simulink library "fam_force_allocation_module_lib"  (R2016b)
settings: Solver=ode45  StartTime=0.0  StopTime=10.0  RelTol=1e-3  EnableMultiTasking=on
values from neighbouring files (symbols this model uses):
  fam_nozzle_orientations = [abp_PM1_nozzle_orientations; abp_PM2_nozzle_orientations]    [fam_force_allocation_module_prep.m]
  fam_P_nozzle_B_B = [abp_PM1_P_nozzle_B_B; abp_PM2_P_nozzle_B_B]    [fam_force_allocation_module_prep.m]
undefined symbols (not defined in the file or in its folder): fam_lookup_thrust_in
libraries: simulink x8, fam_force_allocation_module_lib x2
settings Model: Creator=jfusco1  LastModifiedBy=jfusco1
settings DataIOCC: LimitDataPoints=on  SaveFormat=Array
settings OptimizationCC: LifeSpan=inf
settings DebuggingCC: SolverPrmCheckMsg=warning  AllowSymbolicDim=off  SFUnexpectedBacktrackingDiag=warning  SFNoUnconditionalDefaultTransitionDiag=warning  SFExecutionAtInitializationDiag=none
settings HardwareCC: ProdBitPerPointer=32  ProdBitPerSizeT=32  ProdBitPerPtrDiffT=32  ProdLargestAtomicFloat=None  ProdIntDivRoundTo=Undefined  ProdEndianess=Unspecified  ProdWordSize=32  ProdHWDeviceType=32-bit Generic
settings ModelReferenceCC: PropagateSignalLabelsOutOfModel=off
settings GRTTargetCC: TargetLangStandard=C89/C90 (ANSI)  GeneratePreprocessorConditionals=Disable all
settings ConfigComp: CovMetricSettings=dw  CovHtmlReporting=on  CovSaveCumulativeToWorkspaceVar=on  CovSaveSingleToWorkspaceVar=on  CovExternalEMLEnable=off  CovSFcnEnable=off

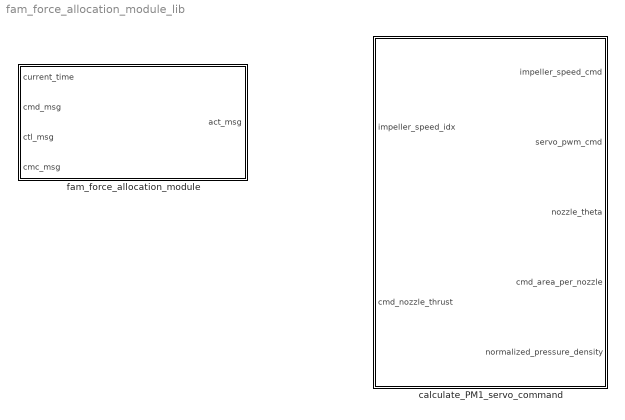
== system fam_force_allocation_module_lib ==
  calculate_PM1_servo_command : Subsystem  mask{impeller_speed_cnt=0, impeller_speeds=0, impeller_speed2pwm=0, impeller_diameter=0, lookup_Cdp=0, lookup_thrust=0, nozzle_widths=0, nozzle_flap_cnt=0, nozzle_flap_length=0, nozzle_in_height=0, nozzle_discharge_coeff=0, nozzle_min_angle=0, nozzle_max_angle=0, nozzle_angle2pwm=0, servo_min_pwm=0, air_density=0}
      mask prompts: impeller_speed_cnt "Number of Speeds"; impeller_speeds "Speeds vs idx"; impeller_speed2pwm "Speed2PWM conversion"; impeller_diameter "Diameter"; lookup_Cdp "Cdp Data"; lookup_thrust "Thrust Breakpoints"; nozzle_widths "Widths"; nozzle_flap_cnt "Flap Count"; nozzle_flap_length "Flap Length"; nozzle_in_height "Intake Height"; nozzle_discharge_coeff "Discharge Coefficients"; nozzle_min_angle "Min Open Angle"; nozzle_max_angle "Max Open Angle"; nozzle_angle2pwm "Angle2PWM conversion"; servo_min_pwm "Minimum PWM"; air_density "Air Density"
      mask DialogControl DescTextVar Prompt: Converts nozzle thrust commands into servo commands
  fam_force_allocation_module : Subsystem

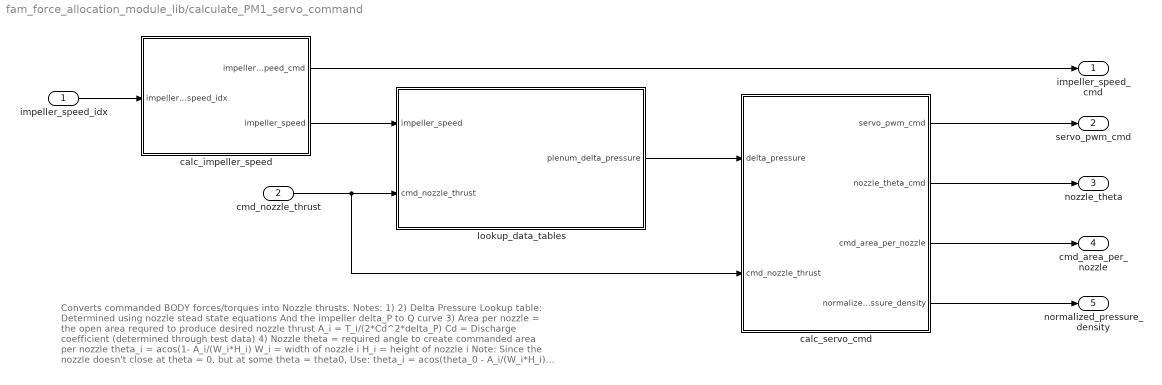
== system fam_force_allocation_module_lib/calculate_PM1_servo_command ==
  note: Converts commanded BODY forces/torques into Nozzle thrusts.
      |
      | Notes:
      | 1)
      | 2) Delta Pressure Lookup table:
      | Determined using nozzle stead state equations
      | And the impeller delta_P to Q curve
      | 3) Area per nozzle = the open area requred to produce desired nozzle thrust
      | A_i = T_i/(2*Cd^2*delta_P)
      | Cd = Discharge coefficient (determined through test data)
      | 4) Nozzle theta = required angle to create commanded area per nozzle
      | theta_i = acos(1- A_i/(W_i*H_i)
      | W_i = width of nozzle i
      | H_i = height of nozzle i
      | Note: Since the nozzle doesn't close at theta = 0, but at some theta = theta0,
      | Use: theta_i = acos(theta_0 - A_i/(W_i*H_i)
      | 5) servo_thetas = commanded theta to each servo
      | theta_si = theta_ni*R
      | R= gear ratio
      | theta_ni = commanded nozzle theta of nozzle 'i'
  impeller_speed_idx : Inport
  cmd_nozzle_thrust : Inport  Port=2
  calc_impeller_speed : Subsystem
  calc_servo_cmd : Subsystem
  lookup_data_tables : Subsystem
  impeller_speed_cmd : Outport
  servo_pwm_cmd : Outport  Port=2
  nozzle_theta : Outport  Port=3
  cmd_area_per_nozzle : Outport  Port=4
  normalized_pressure_density : Outport  Port=5
  wires:
  calc_servo_cmd/4(normalized_pressure_density) -> normalized_pressure_density/1
  calc_servo_cmd/3(cmd_area_per_nozzle) -> cmd_area_per_nozzle/1
  calc_servo_cmd/2(nozzle_theta_cmd) -> nozzle_theta/1
  calc_servo_cmd/1(servo_pwm_cmd) -> servo_pwm_cmd/1
  cmd_nozzle_thrust/1 -> lookup_data_tables/2(cmd_nozzle_thrust), calc_servo_cmd/2(cmd_nozzle_thrust)
  lookup_data_tables/1(plenum_delta_pressure) -> calc_servo_cmd/1(delta_pressure)
  impeller_speed_idx/1 -> calc_impeller_speed/1(impeller_speed_idx)
  calc_impeller_speed/2(impeller_speed) -> lookup_data_tables/1(impeller_speed)
  calc_impeller_speed/1(impeller_speed_cmd) -> impeller_speed_cmd/1

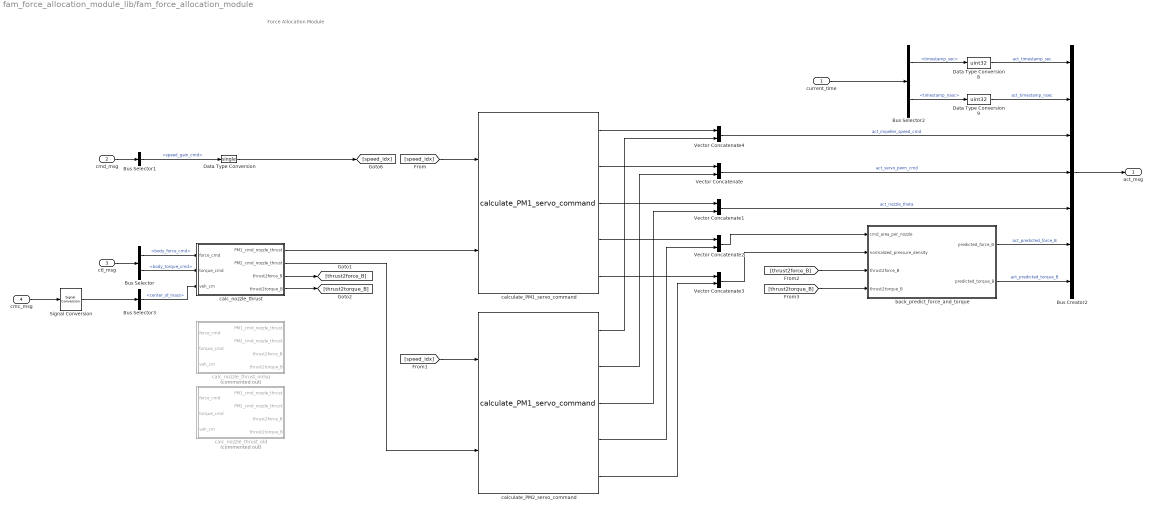
== system fam_force_allocation_module_lib/fam_force_allocation_module ==
  note: Force Allocation Module
  current_time : Inport
  cmd_msg : Inport  Port=2
  ctl_msg : Inport  Port=3
  cmc_msg : Inport  Port=4  OutDataTypeStr=Bus: cmc_msg
  Bus Creator2 : BusCreator  Inputs=7  OutDataTypeStr=Bus: act_msg  NonVirtualBus=on
      settings: InheritFromInputs=off
  Bus Selector : BusSelector  OutputSignals=body_force_cmd,body_torque_cmd
  Bus Selector1 : BusSelector  OutputSignals=speed_gain_cmd
  Bus Selector2 : BusSelector  OutputSignals=timestamp_sec,timestamp_nsec
  Bus Selector3 : BusSelector  OutputSignals=center_of_mass
  Data Type Conversion : DataTypeConversion  OutDataTypeStr=single
  Data Type Conversion8 : DataTypeConversion  OutDataTypeStr=uint32
  Data Type Conversion9 : DataTypeConversion  OutDataTypeStr=uint32
  Signal Conversion : SignalConversion  OverrideOpt=on
  Vector Concatenate{,1..4} (5 alike) : Concatenate
  back_predict_force_and_torque : Subsystem
  calc_nozzle_thrust : Subsystem
  calc_nozzle_thrust_nnlsq : Subsystem  Commented=on
  calc_nozzle_thrust_old : Subsystem  Commented=on
  calculate_PM1_servo_command : fam_force_allocation_module_lib/calculate_PM1_servo_command  impeller_speed_cnt=fam_impeller_speeds_cnt  impeller_speeds=fam_impeller_speeds  impeller_speed2pwm=abp_impeller_speed2pwm  impeller_diameter=abp_impeller_diameter  lookup_Cdp=fam_PM1_lookup_Cdp_data  lookup_thrust=fam_PM1_lookup_thrust_breakpoints  nozzle_widths=abp_PM1_nozzle_widths  nozzle_flap_cnt=abp_nozzle_flap_count  nozzle_flap_length=abp_nozzle_flap_length  nozzle_in_height=abp_nozzle_intake_height  nozzle_discharge_coeff=abp_PM1_discharge_coeff  nozzle_min_angle=abp_nozzle_min_open_angle  nozzle_max_angle=abp_nozzle_max_open_angle  nozzle_angle2pwm=fam_nozzle_angle2pwm  servo_min_pwm=abp_servo_min_PWM  air_density=const_air_density
  calculate_PM2_servo_command : fam_force_allocation_module_lib/calculate_PM1_servo_command  impeller_speed_cnt=fam_impeller_speeds_cnt  impeller_speeds=fam_impeller_speeds  impeller_speed2pwm=abp_impeller_speed2pwm  impeller_diameter=abp_impeller_diameter  lookup_Cdp=fam_PM2_lookup_Cdp_data  lookup_thrust=fam_PM2_lookup_thrust_breakpoints  nozzle_widths=abp_PM2_nozzle_widths  nozzle_flap_cnt=abp_nozzle_flap_count  nozzle_flap_length=abp_nozzle_flap_length  nozzle_in_height=abp_nozzle_intake_height  nozzle_discharge_coeff=abp_PM2_discharge_coeff  nozzle_min_angle=abp_nozzle_min_open_angle  nozzle_max_angle=abp_nozzle_max_open_angle  nozzle_angle2pwm=fam_nozzle_angle2pwm  servo_min_pwm=abp_servo_min_PWM  air_density=const_air_density
  act_msg : Outport
  wires:
  [thrust2torque_B] -> back_predict_force_and_torque/4(thrust2torque_B)
  [thrust2force_B] -> back_predict_force_and_torque/3(thrust2force_B)
  calc_nozzle_thrust/4(thrust2torque_B) -> [thrust2torque_B]
  calc_nozzle_thrust/3(thrust2force_B) -> [thrust2force_B]
  back_predict_force_and_torque/2(predicted_torque_B) -> Bus Creator2/7  "act_predicted_torque_B"
  back_predict_force_and_torque/1(predicted_force_B) -> Bus Creator2/6  "act_predicted_force_B"
  calc_nozzle_thrust/2(PM2_cmd_nozzle_thrust) -> calculate_PM2_servo_command/2
  calc_nozzle_thrust/1(PM1_cmd_nozzle_thrust) -> calculate_PM1_servo_command/2
  [speed_idx] -> calculate_PM2_servo_command/1
  [speed_idx] -> calculate_PM1_servo_command/1
  calculate_PM2_servo_command/5 -> Vector Concatenate3/2
  calculate_PM2_servo_command/4 -> Vector Concatenate2/2
  calculate_PM2_servo_command/3 -> Vector Concatenate1/2
  calculate_PM2_servo_command/2 -> Vector Concatenate/2
  calculate_PM2_servo_command/1 -> Vector Concatenate4/2
  calculate_PM1_servo_command/5 -> Vector Concatenate3/1
  calculate_PM1_servo_command/4 -> Vector Concatenate2/1
  calculate_PM1_servo_command/3 -> Vector Concatenate1/1
  calculate_PM1_servo_command/2 -> Vector Concatenate/1
  calculate_PM1_servo_command/1 -> Vector Concatenate4/1
  Vector Concatenate3/1 -> back_predict_force_and_torque/2(normalized_pressure_density)
  Vector Concatenate2/1 -> back_predict_force_and_torque/1(cmd_area_per_nozzle)
  Vector Concatenate1/1 -> Bus Creator2/5  "act_nozzle_theta"
  Vector Concatenate/1 -> Bus Creator2/4  "act_servo_pwm_cmd"
  Data Type Conversion/1 -> [speed_idx]
  Vector Concatenate4/1 -> Bus Creator2/3  "act_impeller_speed_cmd"
  Data Type Conversion8/1 -> Bus Creator2/1  "act_timestamp_sec"
  Data Type Conversion9/1 -> Bus Creator2/2  "act_timestamp_nsec"
  Bus Selector2/1 -> Data Type Conversion8/1  "<timestamp_sec>"
  Bus Selector2/2 -> Data Type Conversion9/1  "<timestamp_nsec>"
  Bus Creator2/1 -> act_msg/1
  current_time/1 -> Bus Selector2/1
  Bus Selector/2 -> calc_nozzle_thrust/2(torque_cmd)  "<body_torque_cmd>"
  Bus Selector/1 -> calc_nozzle_thrust/1(force_cmd)  "<body_force_cmd>"
  ctl_msg/1 -> Bus Selector/1
  cmd_msg/1 -> Bus Selector1/1
  Bus Selector1/1 -> Data Type Conversion/1  "<speed_gain_cmd>"
  Signal Conversion/1 -> Bus Selector3/1
  Bus Selector3/1 -> calc_nozzle_thrust/3(veh_cm)  "<center_of_mass>"
  cmc_msg/1 -> Signal Conversion/1

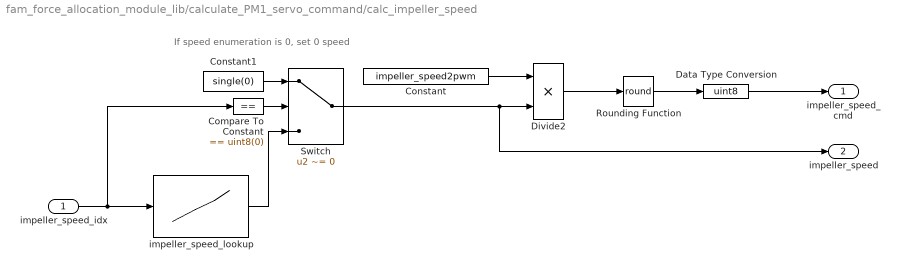
== system fam_force_allocation_module_lib/calculate_PM1_servo_command/calc_impeller_speed ==
  note: If speed enumeration is 0, set 0 speed
  impeller_speed_idx : Inport
  Compare To Constant : simulink/Logic and Bit Operations/Compare To Constant  relop===  const=uint8(0)  OutDataTypeStr=boolean
  Constant : Constant  Value=impeller_speed2pwm
  Constant1 : Constant  Value=single(0)
  Data Type Conversion : DataTypeConversion  OutDataTypeStr=uint8
  Divide2 : Product  Inputs=**
  Rounding Function : Rounding  Operator=round
  Switch : Switch  Criteria=u2 ~= 0
  impeller_speed_lookup : Lookup_n-D  NumberOfTableDimensions=1  BreakpointsForDimension1=[1:impeller_speed_cnt]  BreakpointsForDimension2=fam_lookup_thrust_in  BeginIndexSearchUsingPreviousIndexResult=on  Table=impeller_speeds  InterpMethod=Nearest  ExtrapMethod=Clip  InternalRulePriority=Speed  RndMeth=Simplest  InputSameDT=on
      settings: AttributesFormatString=|
      | Data Table: %<Table>
      | #dim: %<NumberOfTableDimensions>
      | BP1: %<BreakpointsForDimension1>
  impeller_speed_cmd : Outport
  impeller_speed : Outport  Port=2
  wires:
  Data Type Conversion/1 -> impeller_speed_cmd/1
  Rounding Function/1 -> Data Type Conversion/1
  Divide2/1 -> Rounding Function/1
  Constant/1 -> Divide2/1
  impeller_speed_idx/1 -> impeller_speed_lookup/1, Compare To Constant/1
  Switch/1 -> impeller_speed/1, Divide2/2
  Compare To Constant/1 -> Switch/2
  Constant1/1 -> Switch/1
  impeller_speed_lookup/1 -> Switch/3

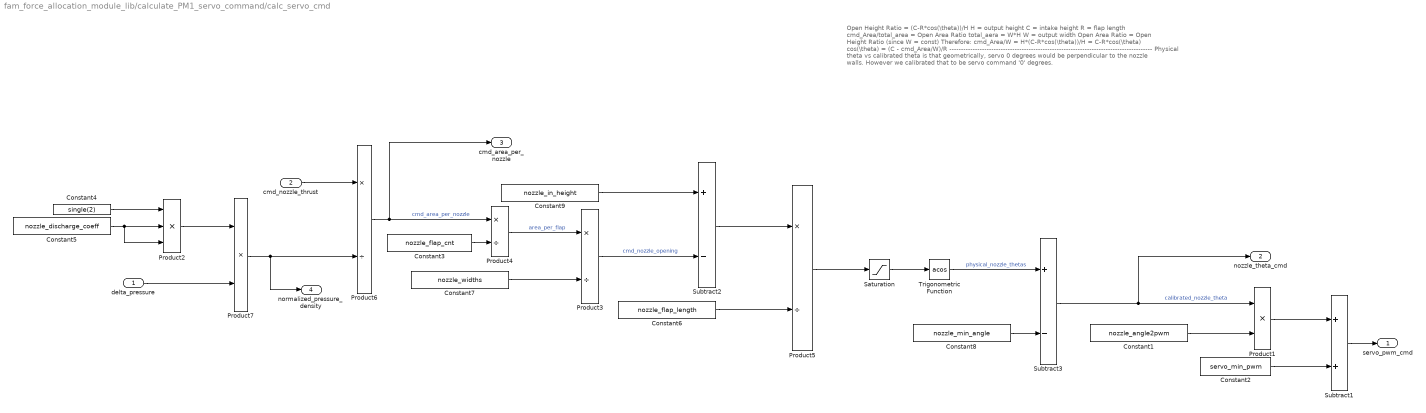
== system fam_force_allocation_module_lib/calculate_PM1_servo_command/calc_servo_cmd ==
  note: Open Height Ratio = (C-R*cos(\theta))/H
      | 	H = output height
      | 	C = intake height
      | 	R = flap length
      |
      | cmd_Area/total_area = Open Area Ratio
      | 	total_aera = W*H
      | 	W = output width
      |
      | Open Area Ratio = Open Height Ratio (since W = const)
      |
      | Therefore:
      | cmd_Area/W = H*(C-R*cos(\theta))/H = C-R*cos(\theta)
      | cos(\theta) = (C - cmd_Area/W)/R
      |
      | ---------------------------------------------------------------------------------------
      |
      | Physical theta vs calibrated theta is that geometrically, servo 0 degrees would be perpendicular to the nozzle walls.
      | 	However we calibrated that to be servo command '0' degrees.
  delta_pressure : Inport
  cmd_nozzle_thrust : Inport  Port=2
  Constant1 : Constant  Value=nozzle_angle2pwm
  Constant2 : Constant  Value=servo_min_pwm
  Constant3 : Constant  Value=nozzle_flap_cnt
  Constant4 : Constant  Value=single(2)
  Constant5 : Constant  Value=nozzle_discharge_coeff
  Constant6 : Constant  Value=nozzle_flap_length
  Constant7 : Constant  Value=nozzle_widths
  Constant8 : Constant  Value=nozzle_min_angle
  Constant9 : Constant  Value=nozzle_in_height
  Product1 : Product  Inputs=**
  Product2 : Product  Inputs=***
  Product{3..6} (4 alike) : Product  Inputs=*/
  Product7 : Product  Inputs=**
  Saturation : Saturate  UpperLimit=cos(nozzle_min_angle)  LowerLimit=cos(nozzle_max_angle)
      settings: AttributesFormatString=|
      | Max: %<UpperLimit>
      | Min: %<LowerLimit>
  Subtract1 : Sum
  Subtract2 : Sum  Inputs=+-
  Subtract3 : Sum  Inputs=+-
  Trigonometric Function : Trigonometry  Operator=acos
  servo_pwm_cmd : Outport
  nozzle_theta_cmd : Outport  Port=2
  cmd_area_per_nozzle : Outport  Port=3
  normalized_pressure_density : Outport  Port=4
  wires:
  Saturation/1 -> Trigonometric Function/1
  Product5/1 -> Saturation/1
  Product6/1 -> cmd_area_per_nozzle/1, Product4/1  "cmd_area_per_nozzle"
  Constant4/1 -> Product2/1
  Product1/1 -> Subtract1/1
  Subtract1/1 -> servo_pwm_cmd/1
  Constant1/1 -> Product1/2
  Constant2/1 -> Subtract1/2
  Constant5/1 -> Product2/3, Product2/2
  delta_pressure/1 -> Product7/2
  Product2/1 -> Product7/1
  Constant7/1 -> Product3/2
  Product3/1 -> Subtract2/2  "cmd_nozzle_opening"
  Constant9/1 -> Subtract2/1
  Constant6/1 -> Product5/2
  Subtract2/1 -> Product5/1
  Constant3/1 -> Product4/2
  Product4/1 -> Product3/1  "area_per_flap"
  Product7/1 -> Product6/2, normalized_pressure_density/1
  cmd_nozzle_thrust/1 -> Product6/1
  Trigonometric Function/1 -> Subtract3/1  "physical_nozzle_thetas"
  Subtract3/1 -> Product1/1, nozzle_theta_cmd/1  "calibrated_nozzle_theta"
  Constant8/1 -> Subtract3/2

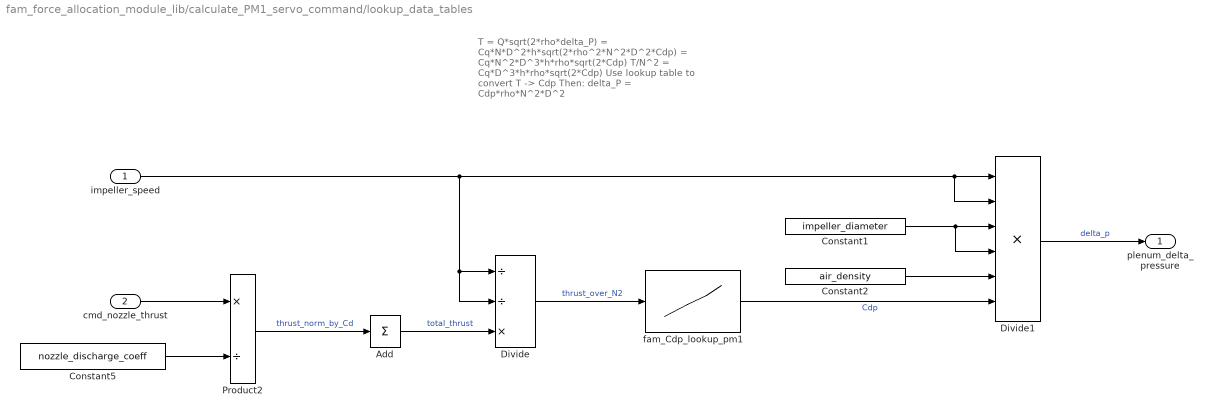
== system fam_force_allocation_module_lib/calculate_PM1_servo_command/lookup_data_tables ==
  note: T = Q*sqrt(2*rho*delta_P)
      | 	= Cq*N*D^2*h*sqrt(2*rho^2*N^2*D^2*Cdp)
      | 	= Cq*N^2*D^3*h*rho*sqrt(2*Cdp)
      | T/N^2 = Cq*D^3*h*rho*sqrt(2*Cdp)
      |
      | Use lookup table to convert T -> Cdp
      | Then: delta_P = Cdp*rho*N^2*D^2
  impeller_speed : Inport
  cmd_nozzle_thrust : Inport  Port=2
  Add : Sum  Inputs=+
  Constant1 : Constant  Value=impeller_diameter
  Constant2 : Constant  Value=air_density
  Constant5 : Constant  Value=nozzle_discharge_coeff
  Divide : Product  Inputs=//*
  Divide1 : Product  Inputs=******
  Product2 : Product  Inputs=*/
  fam_Cdp_lookup_pm1 : Lookup_n-D  NumberOfTableDimensions=1  BreakpointsForDimension1=lookup_thrust  BreakpointsForDimension2=fam_lookup_thrust_in  BeginIndexSearchUsingPreviousIndexResult=on  Table=lookup_Cdp  ExtrapMethod=Clip  UseLastTableValue=on  InternalRulePriority=Speed  RndMeth=Simplest  InputSameDT=on
      settings: AttributesFormatString=|
      | Data Table: %<Table>
      | #dim: %<NumberOfTableDimensions>
      | BP1: %<BreakpointsForDimension1>
  plenum_delta_pressure : Outport
  wires:
  Add/1 -> Divide/3  "total_thrust"
  Constant5/1 -> Product2/2
  cmd_nozzle_thrust/1 -> Product2/1
  Product2/1 -> Add/1  "thrust_norm_by_Cd"
  Divide/1 -> fam_Cdp_lookup_pm1/1  "thrust_over_N2"
  fam_Cdp_lookup_pm1/1 -> Divide1/6  "Cdp"
  Constant1/1 -> Divide1/4, Divide1/3
  impeller_speed/1 -> Divide1/2, Divide1/1, Divide/1, Divide/2
  Constant2/1 -> Divide1/5
  Divide1/1 -> plenum_delta_pressure/1  "delta_p"

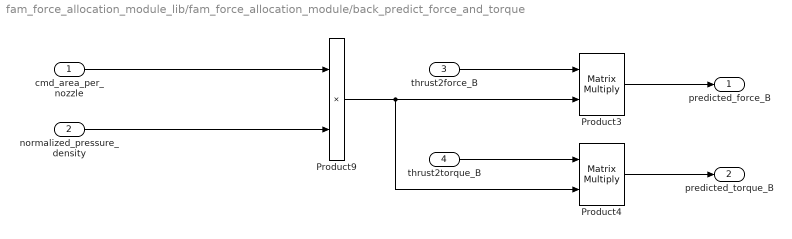
== system fam_force_allocation_module_lib/fam_force_allocation_module/back_predict_force_and_torque ==
  cmd_area_per_nozzle : Inport
  normalized_pressure_density : Inport  Port=2
  thrust2force_B : Inport  Port=3
  thrust2torque_B : Inport  Port=4
  Product3 : Product  Multiplication=Matrix(*)
  Product4 : Product  Multiplication=Matrix(*)
  Product9 : Product  Inputs=**
  predicted_force_B : Outport
  predicted_torque_B : Outport  Port=2
  wires:
  normalized_pressure_density/1 -> Product9/2
  cmd_area_per_nozzle/1 -> Product9/1
  thrust2force_B/1 -> Product3/1
  Product9/1 -> Product3/2, Product4/2
  thrust2torque_B/1 -> Product4/1
  Product3/1 -> predicted_force_B/1
  Product4/1 -> predicted_torque_B/1

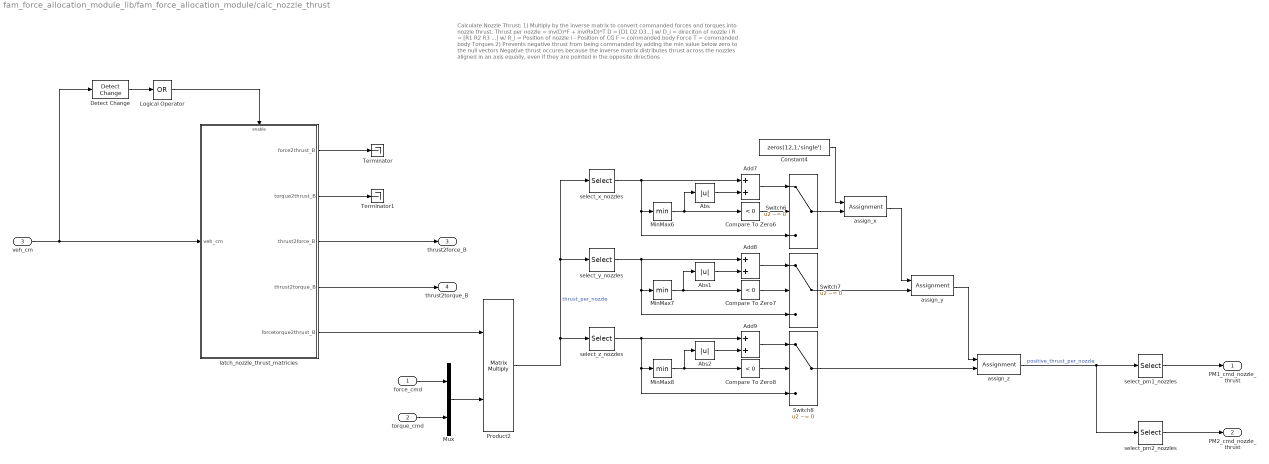
== system fam_force_allocation_module_lib/fam_force_allocation_module/calc_nozzle_thrust ==
  note: Calculate Nozzle Thrust:
      | 1) Multiply by the inverse matrix to convert commanded forces and torques into nozzle thrust.
      | Thrust per nozzle = inv(D)*F + inv(RxD)*T
      | D = [D1 D2 D3...] w/ D_i = direciton of nozzle i
      | R = [R1 R2 R3 ...] w/ R_i = Position of nozzle i - Position of CG
      | F = commanded body Force
      | T = commanded body Torques
      | 2) Prevents negative thrust from being commanded by adding the min value below zero to the null vectors
      | Negative thrust occures because the inverse matrix distributes thrust across the nozzles aligned in an axis equally, even if they are pointed in the opposite directions
  force_cmd : Inport
  torque_cmd : Inport  Port=2
  veh_cm : Inport  Port=3
  Abs : Abs
  Abs1 : Abs
  Abs2 : Abs
  Add7 : Sum
  Add8 : Sum
  Add9 : Sum
  Compare To Zero6 : simulink/Logic and Bit Operations/Compare To Zero  relop=<  OutDataTypeStr=boolean
  Compare To Zero7 : simulink/Logic and Bit Operations/Compare To Zero  relop=<  OutDataTypeStr=boolean
  Compare To Zero8 : simulink/Logic and Bit Operations/Compare To Zero  relop=<  OutDataTypeStr=boolean
  Constant4 : Constant  Value=zeros(12,1,'single')
  Detect Change : simulink/Logic and Bit Operations/Detect Change  vinit=inf  OutDataTypeStr=boolean
  Logical Operator : Logic  Operator=OR  Inputs=1  AllPortsSameDT=off  OutDataTypeStr=boolean
  MinMax6 : MinMax
  MinMax7 : MinMax
  MinMax8 : MinMax
  Mux : Mux  Inputs=2
  Product2 : Product  Multiplication=Matrix(*)
  Switch6 : Switch  Criteria=u2 ~= 0
  Switch7 : Switch  Criteria=u2 ~= 0
  Switch8 : Switch  Criteria=u2 ~= 0
  Terminator : Terminator
  Terminator1 : Terminator
  assign_x : Assignment  DiagnosticForDimensions=Warning  IndexOptions=Index vector (dialog)  Indices=fam_nozzle_x_dir  OutputSizes=1
      settings: AttributesFormatString=Selects: %<Indices>
  assign_y : Assignment  DiagnosticForDimensions=Warning  IndexOptions=Index vector (dialog)  Indices=fam_nozzle_y_dir  OutputSizes=1
      settings: AttributesFormatString=Selects: %<Indices>
  assign_z : Assignment  DiagnosticForDimensions=Warning  IndexOptions=Index vector (dialog)  Indices=fam_nozzle_z_dir  OutputSizes=1
      settings: AttributesFormatString=Selects: %<Indices>
  latch_nozzle_thrust_matricies : Subsystem
  select_pm1_nozzles : Selector  InputPortWidth=12  IndexOptions=Index vector (dialog)  Indices=fam_nozzle_pm1  OutputSizes=1
      settings: AttributesFormatString=|
      | Input Width: %<InputPortWidth>
      | Selects: %<Indices>
  select_pm2_nozzles : Selector  InputPortWidth=12  IndexOptions=Index vector (dialog)  Indices=fam_nozzle_pm2  OutputSizes=1
      settings: AttributesFormatString=|
      | Input Width: %<InputPortWidth>
      | Selects: %<Indices>
  select_x_nozzles : Selector  InputPortWidth=12  IndexOptions=Index vector (dialog)  Indices=fam_nozzle_x_dir  OutputSizes=1
      settings: AttributesFormatString=|
      | Input Width: %<InputPortWidth>
      | Selects: %<Indices>
  select_y_nozzles : Selector  InputPortWidth=12  IndexOptions=Index vector (dialog)  Indices=fam_nozzle_y_dir  OutputSizes=1
      settings: AttributesFormatString=|
      | Input Width: %<InputPortWidth>
      | Selects: %<Indices>
  select_z_nozzles : Selector  InputPortWidth=12  IndexOptions=Index vector (dialog)  Indices=fam_nozzle_z_dir  OutputSizes=1
      settings: AttributesFormatString=|
      | Input Width: %<InputPortWidth>
      | Selects: %<Indices>
  PM1_cmd_nozzle_thrust : Outport
  PM2_cmd_nozzle_thrust : Outport  Port=2
  thrust2force_B : Outport  Port=3
  thrust2torque_B : Outport  Port=4
  wires:
  veh_cm/1 -> Detect Change/1, latch_nozzle_thrust_matricies/1(veh_cm)
  assign_z/1 -> select_pm2_nozzles/1, select_pm1_nozzles/1  "positive_thrust_per_nozzle"
  select_x_nozzles/1 -> Switch6/3, MinMax6/1, Add7/1
  MinMax6/1 -> Abs/1, Compare To Zero6/1
  Compare To Zero6/1 -> Switch6/2
  Add7/1 -> Switch6/1
  Compare To Zero7/1 -> Switch7/2
  Add8/1 -> Switch7/1
  Compare To Zero8/1 -> Switch8/2
  Add9/1 -> Switch8/1
  Switch6/1 -> assign_x/2
  Switch7/1 -> assign_y/2
  Switch8/1 -> assign_z/2
  assign_y/1 -> assign_z/1
  assign_x/1 -> assign_y/1
  Constant4/1 -> assign_x/1
  Abs/1 -> Add7/2
  select_y_nozzles/1 -> Add8/1, MinMax7/1, Switch7/3
  MinMax7/1 -> Compare To Zero7/1, Abs1/1
  Abs1/1 -> Add8/2
  select_z_nozzles/1 -> Add9/1, Switch8/3, MinMax8/1
  MinMax8/1 -> Compare To Zero8/1, Abs2/1
  Abs2/1 -> Add9/2
  Product2/1 -> select_x_nozzles/1, select_y_nozzles/1, select_z_nozzles/1  "thrust_per_nozzle"
  select_pm2_nozzles/1 -> PM2_cmd_nozzle_thrust/1
  select_pm1_nozzles/1 -> PM1_cmd_nozzle_thrust/1
  latch_nozzle_thrust_matricies/4(thrust2torque_B) -> thrust2torque_B/1
  latch_nozzle_thrust_matricies/3(thrust2force_B) -> thrust2force_B/1
  force_cmd/1 -> Mux/1
  torque_cmd/1 -> Mux/2
  Mux/1 -> Product2/2
  latch_nozzle_thrust_matricies/5(forcetorque2thrust_B) -> Product2/1
  latch_nozzle_thrust_matricies/1(force2thrust_B) -> Terminator/1
  latch_nozzle_thrust_matricies/2(torque2thrust_B) -> Terminator1/1
  Detect Change/1 -> Logical Operator/1
  Logical Operator/1 -> latch_nozzle_thrust_matricies/Enable

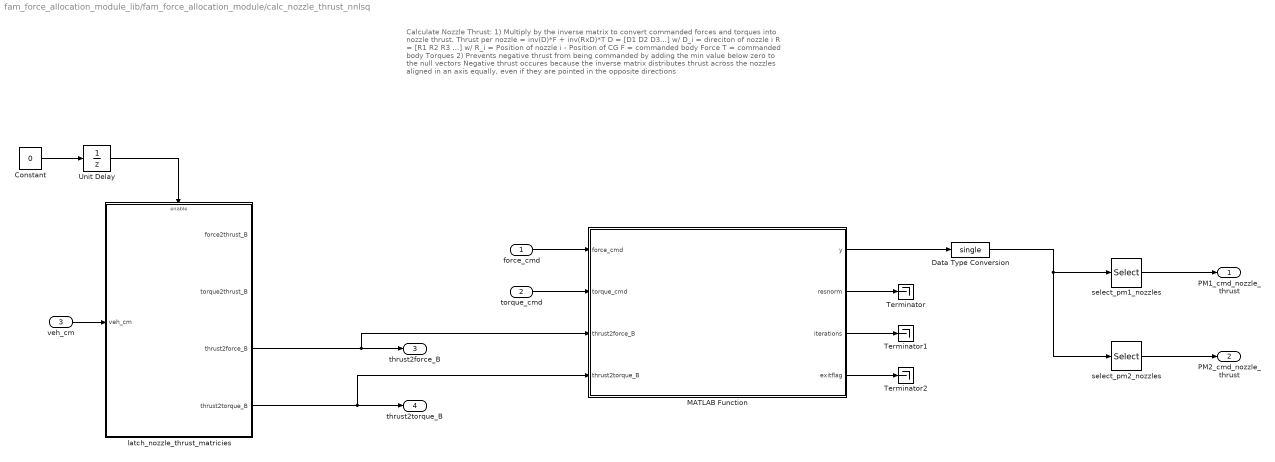
== system fam_force_allocation_module_lib/fam_force_allocation_module/calc_nozzle_thrust_nnlsq ==
  note: Calculate Nozzle Thrust:
      | 1) Multiply by the inverse matrix to convert commanded forces and torques into nozzle thrust.
      | Thrust per nozzle = inv(D)*F + inv(RxD)*T
      | D = [D1 D2 D3...] w/ D_i = direciton of nozzle i
      | R = [R1 R2 R3 ...] w/ R_i = Position of nozzle i - Position of CG
      | F = commanded body Force
      | T = commanded body Torques
      | 2) Prevents negative thrust from being commanded by adding the min value below zero to the null vectors
      | Negative thrust occures because the inverse matrix distributes thrust across the nozzles aligned in an axis equally, even if they are pointed in the opposite directions
  force_cmd : Inport
  torque_cmd : Inport  Port=2
  veh_cm : Inport  Port=3
  Constant : Constant  Value=0
  Data Type Conversion : DataTypeConversion  OutDataTypeStr=single
  MATLAB Function : MATLAB Function  TreatAsAtomicUnit=on
  Terminator : Terminator
  Terminator1 : Terminator
  Terminator2 : Terminator
  Unit Delay : UnitDelay  InitialCondition=1  SampleTime=-1
      settings: AttributesFormatString=IC: %<InitialCondition>
  latch_nozzle_thrust_matricies : Subsystem
  select_pm1_nozzles : Selector  InputPortWidth=12  IndexOptions=Index vector (dialog)  Indices=fam_nozzle_pm1  OutputSizes=1
      settings: AttributesFormatString=|
      | Input Width: %<InputPortWidth>
      | Selects: %<Indices>
  select_pm2_nozzles : Selector  InputPortWidth=12  IndexOptions=Index vector (dialog)  Indices=fam_nozzle_pm2  OutputSizes=1
      settings: AttributesFormatString=|
      | Input Width: %<InputPortWidth>
      | Selects: %<Indices>
  PM1_cmd_nozzle_thrust : Outport
  PM2_cmd_nozzle_thrust : Outport  Port=2
  thrust2force_B : Outport  Port=3
  thrust2torque_B : Outport  Port=4
  wires:
  Constant/1 -> Unit Delay/1
  latch_nozzle_thrust_matricies/3(thrust2force_B) -> MATLAB Function/3(thrust2force_B), thrust2force_B/1
  latch_nozzle_thrust_matricies/4(thrust2torque_B) -> MATLAB Function/4(thrust2torque_B), thrust2torque_B/1
  Unit Delay/1 -> latch_nozzle_thrust_matricies/Enable
  select_pm1_nozzles/1 -> PM1_cmd_nozzle_thrust/1
  select_pm2_nozzles/1 -> PM2_cmd_nozzle_thrust/1
  veh_cm/1 -> latch_nozzle_thrust_matricies/1(veh_cm)
  MATLAB Function/1(y) -> Data Type Conversion/1
  torque_cmd/1 -> MATLAB Function/2(torque_cmd)
  force_cmd/1 -> MATLAB Function/1(force_cmd)
  Data Type Conversion/1 -> select_pm2_nozzles/1, select_pm1_nozzles/1
  MATLAB Function/2(resnorm) -> Terminator/1
  MATLAB Function/3(iterations) -> Terminator1/1
  MATLAB Function/4(exitflag) -> Terminator2/1

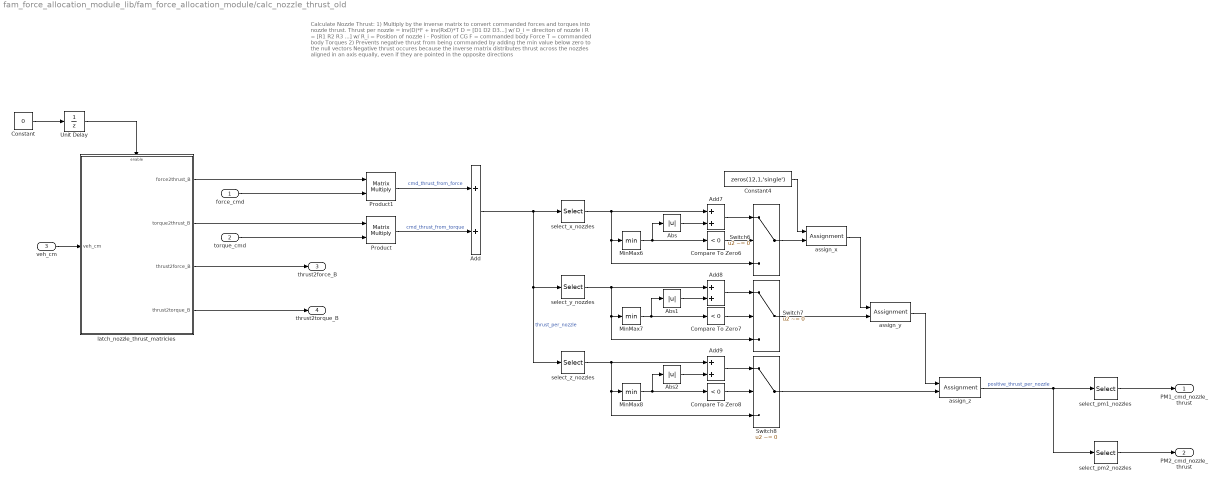
== system fam_force_allocation_module_lib/fam_force_allocation_module/calc_nozzle_thrust_old ==
  note: Calculate Nozzle Thrust:
      | 1) Multiply by the inverse matrix to convert commanded forces and torques into nozzle thrust.
      | Thrust per nozzle = inv(D)*F + inv(RxD)*T
      | D = [D1 D2 D3...] w/ D_i = direciton of nozzle i
      | R = [R1 R2 R3 ...] w/ R_i = Position of nozzle i - Position of CG
      | F = commanded body Force
      | T = commanded body Torques
      | 2) Prevents negative thrust from being commanded by adding the min value below zero to the null vectors
      | Negative thrust occures because the inverse matrix distributes thrust across the nozzles aligned in an axis equally, even if they are pointed in the opposite directions
  force_cmd : Inport
  torque_cmd : Inport  Port=2
  veh_cm : Inport  Port=3
  Abs : Abs
  Abs1 : Abs
  Abs2 : Abs
  Add{,7..9} (4 alike) : Sum
  Compare To Zero6 : simulink/Logic and Bit Operations/Compare To Zero  relop=<  OutDataTypeStr=boolean
  Compare To Zero7 : simulink/Logic and Bit Operations/Compare To Zero  relop=<  OutDataTypeStr=boolean
  Compare To Zero8 : simulink/Logic and Bit Operations/Compare To Zero  relop=<  OutDataTypeStr=boolean
  Constant : Constant  Value=0
  Constant4 : Constant  Value=zeros(12,1,'single')
  MinMax6 : MinMax
  MinMax7 : MinMax
  MinMax8 : MinMax
  Product : Product  Multiplication=Matrix(*)
  Product1 : Product  Multiplication=Matrix(*)
  Switch6 : Switch  Criteria=u2 ~= 0
  Switch7 : Switch  Criteria=u2 ~= 0
  Switch8 : Switch  Criteria=u2 ~= 0
  Unit Delay : UnitDelay  InitialCondition=1  SampleTime=-1
      settings: AttributesFormatString=IC: %<InitialCondition>
  assign_x : Assignment  DiagnosticForDimensions=Warning  IndexOptions=Index vector (dialog)  Indices=fam_nozzle_x_dir  OutputSizes=1
      settings: AttributesFormatString=Selects: %<Indices>
  assign_y : Assignment  DiagnosticForDimensions=Warning  IndexOptions=Index vector (dialog)  Indices=fam_nozzle_y_dir  OutputSizes=1
      settings: AttributesFormatString=Selects: %<Indices>
  assign_z : Assignment  DiagnosticForDimensions=Warning  IndexOptions=Index vector (dialog)  Indices=fam_nozzle_z_dir  OutputSizes=1
      settings: AttributesFormatString=Selects: %<Indices>
  latch_nozzle_thrust_matricies : Subsystem
  select_pm1_nozzles : Selector  InputPortWidth=12  IndexOptions=Index vector (dialog)  Indices=fam_nozzle_pm1  OutputSizes=1
      settings: AttributesFormatString=|
      | Input Width: %<InputPortWidth>
      | Selects: %<Indices>
  select_pm2_nozzles : Selector  InputPortWidth=12  IndexOptions=Index vector (dialog)  Indices=fam_nozzle_pm2  OutputSizes=1
      settings: AttributesFormatString=|
      | Input Width: %<InputPortWidth>
      | Selects: %<Indices>
  select_x_nozzles : Selector  InputPortWidth=12  IndexOptions=Index vector (dialog)  Indices=fam_nozzle_x_dir  OutputSizes=1
      settings: AttributesFormatString=|
      | Input Width: %<InputPortWidth>
      | Selects: %<Indices>
  select_y_nozzles : Selector  InputPortWidth=12  IndexOptions=Index vector (dialog)  Indices=fam_nozzle_y_dir  OutputSizes=1
      settings: AttributesFormatString=|
      | Input Width: %<InputPortWidth>
      | Selects: %<Indices>
  select_z_nozzles : Selector  InputPortWidth=12  IndexOptions=Index vector (dialog)  Indices=fam_nozzle_z_dir  OutputSizes=1
      settings: AttributesFormatString=|
      | Input Width: %<InputPortWidth>
      | Selects: %<Indices>
  PM1_cmd_nozzle_thrust : Outport
  PM2_cmd_nozzle_thrust : Outport  Port=2
  thrust2force_B : Outport  Port=3
  thrust2torque_B : Outport  Port=4
  wires:
  Constant/1 -> Unit Delay/1
  latch_nozzle_thrust_matricies/3(thrust2force_B) -> thrust2force_B/1
  latch_nozzle_thrust_matricies/4(thrust2torque_B) -> thrust2torque_B/1
  Unit Delay/1 -> latch_nozzle_thrust_matricies/Enable
  select_pm1_nozzles/1 -> PM1_cmd_nozzle_thrust/1
  select_pm2_nozzles/1 -> PM2_cmd_nozzle_thrust/1
  Add/1 -> select_x_nozzles/1, select_z_nozzles/1, select_y_nozzles/1  "thrust_per_nozzle"
  Abs2/1 -> Add9/2
  MinMax8/1 -> Abs2/1, Compare To Zero8/1
  select_z_nozzles/1 -> MinMax8/1, Switch8/3, Add9/1
  Abs1/1 -> Add8/2
  MinMax7/1 -> Abs1/1, Compare To Zero7/1
  select_y_nozzles/1 -> Switch7/3, MinMax7/1, Add8/1
  Abs/1 -> Add7/2
  Constant4/1 -> assign_x/1
  assign_x/1 -> assign_y/1
  assign_y/1 -> assign_z/1
  Switch8/1 -> assign_z/2
  Switch7/1 -> assign_y/2
  Switch6/1 -> assign_x/2
  Add9/1 -> Switch8/1
  Compare To Zero8/1 -> Switch8/2
  Add8/1 -> Switch7/1
  Compare To Zero7/1 -> Switch7/2
  Add7/1 -> Switch6/1
  Compare To Zero6/1 -> Switch6/2
  MinMax6/1 -> Compare To Zero6/1, Abs/1
  select_x_nozzles/1 -> Add7/1, MinMax6/1, Switch6/3
  Product1/1 -> Add/1  "cmd_thrust_from_force"
  latch_nozzle_thrust_matricies/2(torque2thrust_B) -> Product/1
  latch_nozzle_thrust_matricies/1(force2thrust_B) -> Product1/1
  Product/1 -> Add/2  "cmd_thrust_from_torque"
  torque_cmd/1 -> Product/2
  force_cmd/1 -> Product1/2
  assign_z/1 -> select_pm1_nozzles/1, select_pm2_nozzles/1  "positive_thrust_per_nozzle"
  veh_cm/1 -> latch_nozzle_thrust_matricies/1(veh_cm)

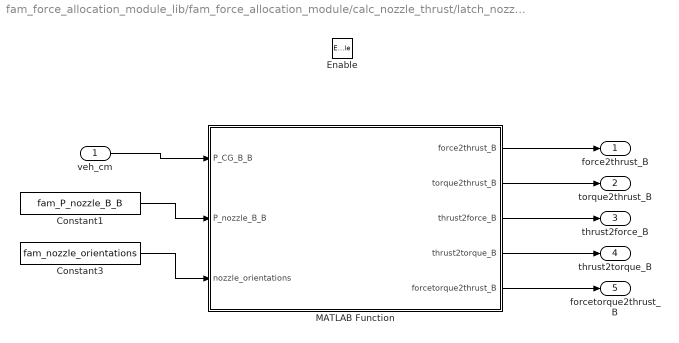
== system fam_force_allocation_module_lib/fam_force_allocation_module/calc_nozzle_thrust/latch_nozzle_thrust_matricies ==
  veh_cm : Inport
  Enable : EnablePort  ZeroCross=off
  Constant1 : Constant  Value=fam_P_nozzle_B_B
  Constant3 : Constant  Value=fam_nozzle_orientations
  MATLAB Function : MATLAB Function  TreatAsAtomicUnit=on
  force2thrust_B : Outport
  torque2thrust_B : Outport  Port=2
  thrust2force_B : Outport  Port=3
  thrust2torque_B : Outport  Port=4
  forcetorque2thrust_B : Outport  Port=5
  wires:
  Constant1/1 -> MATLAB Function/2(P_nozzle_B_B)
  veh_cm/1 -> MATLAB Function/1(P_CG_B_B)
  Constant3/1 -> MATLAB Function/3(nozzle_orientations)
  MATLAB Function/2(torque2thrust_B) -> torque2thrust_B/1
  MATLAB Function/1(force2thrust_B) -> force2thrust_B/1
  MATLAB Function/3(thrust2force_B) -> thrust2force_B/1
  MATLAB Function/4(thrust2torque_B) -> thrust2torque_B/1
  MATLAB Function/5(forcetorque2thrust_B) -> forcetorque2thrust_B/1

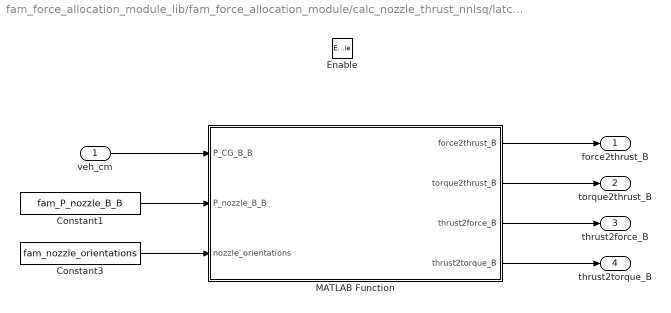
== system fam_force_allocation_module_lib/fam_force_allocation_module/calc_nozzle_thrust_nnlsq/latch_nozzle_thrust_matricies ==
  veh_cm : Inport
  Enable : EnablePort  ZeroCross=off
  Constant1 : Constant  Value=fam_P_nozzle_B_B
  Constant3 : Constant  Value=fam_nozzle_orientations
  MATLAB Function : MATLAB Function  TreatAsAtomicUnit=on
  force2thrust_B : Outport
  torque2thrust_B : Outport  Port=2
  thrust2force_B : Outport  Port=3
  thrust2torque_B : Outport  Port=4
  wires:
  MATLAB Function/4(thrust2torque_B) -> thrust2torque_B/1
  MATLAB Function/3(thrust2force_B) -> thrust2force_B/1
  MATLAB Function/1(force2thrust_B) -> force2thrust_B/1
  MATLAB Function/2(torque2thrust_B) -> torque2thrust_B/1
  Constant3/1 -> MATLAB Function/3(nozzle_orientations)
  veh_cm/1 -> MATLAB Function/1(P_CG_B_B)
  Constant1/1 -> MATLAB Function/2(P_nozzle_B_B)

== system fam_force_allocation_module_lib/fam_force_allocation_module/calc_nozzle_thrust_old/latch_nozzle_thrust_matricies ==
  veh_cm : Inport
  Enable : EnablePort  ZeroCross=off
  Constant1 : Constant  Value=fam_P_nozzle_B_B
  Constant3 : Constant  Value=fam_nozzle_orientations
  MATLAB Function : MATLAB Function  TreatAsAtomicUnit=on
  force2thrust_B : Outport
  torque2thrust_B : Outport  Port=2
  thrust2force_B : Outport  Port=3
  thrust2torque_B : Outport  Port=4
  wires:
  MATLAB Function/4(thrust2torque_B) -> thrust2torque_B/1
  MATLAB Function/3(thrust2force_B) -> thrust2force_B/1
  MATLAB Function/1(force2thrust_B) -> force2thrust_B/1
  MATLAB Function/2(torque2thrust_B) -> torque2thrust_B/1
  Constant3/1 -> MATLAB Function/3(nozzle_orientations)
  veh_cm/1 -> MATLAB Function/1(P_CG_B_B)
  Constant1/1 -> MATLAB Function/2(P_nozzle_B_B)

== matlab function fam_force_allocation_module_lib/fam_force_allocation_module/calc_nozzle_thrust_old/latch_nozzle_thrust_matricies/MATLAB Function ==
  data: P_CG_B_B input size=[1 3]; force2thrust_B output; torque2thrust_B output; P_nozzle_B_B input; nozzle_orientations input; thrust2force_B output; thrust2torque_B output
function [force2thrust_B, torque2thrust_B, thrust2force_B, thrust2torque_B] = calc_thrust_matricies(P_CG_B_B, P_nozzle_B_B, nozzle_orientations)
%#codegen

%NOTE: if number of nozzles change, must change this hard coded '12' below
nozzle_moment_arm       = P_nozzle_B_B - repmat(P_CG_B_B,12,1);                 %[m] Distance from nozzles to CG

thrust2torque_B         = -cross(nozzle_moment_arm, nozzle_orientations,2)';   %[-] Converts a nozzle thrust into resulting body torques
torque2thrust_B         = pinv(thrust2torque_B);                               %[-] Converts body torques into nozzle thrust
thrust2force_B          = -nozzle_orientations';                               %[-] Converts a nozzle thrust into resulting body forces
force2thrust_B          = pinv(thrust2force_B);                                %[-] Converts body forces into nozzle thrust

end

== matlab function fam_force_allocation_module_lib/fam_force_allocation_module/calc_nozzle_thrust_nnlsq/latch_nozzle_thrust_matricies/MATLAB Function ==
  data: P_CG_B_B input size=[1 3]; force2thrust_B output; torque2thrust_B output; P_nozzle_B_B input; nozzle_orientations input; thrust2force_B output; thrust2torque_B output
function [force2thrust_B, torque2thrust_B, thrust2force_B, thrust2torque_B] = calc_thrust_matricies(P_CG_B_B, P_nozzle_B_B, nozzle_orientations)
%#codegen

%NOTE: if number of nozzles change, must change this hard coded '12' below
nozzle_moment_arm       = P_nozzle_B_B - repmat(P_CG_B_B,12,1);                 %[m] Distance from nozzles to CG

thrust2torque_B         = -cross(nozzle_moment_arm, nozzle_orientations,2)';   %[-] Converts a nozzle thrust into resulting body torques
torque2thrust_B         = pinv(thrust2torque_B);                               %[-] Converts body torques into nozzle thrust
thrust2force_B          = -nozzle_orientations';                               %[-] Converts a nozzle thrust into resulting body forces
force2thrust_B          = pinv(thrust2force_B);                                %[-] Converts body forces into nozzle thrust

end

== matlab function fam_force_allocation_module_lib/fam_force_allocation_module/calc_nozzle_thrust_nnlsq/MATLAB Function ==
  data: force_cmd input; y output; torque_cmd input; thrust2force_B input; thrust2torque_B input; resnorm output; iterations output; exitflag output
function [y, resnorm, iterations, exitflag] = fcn(force_cmd, torque_cmd, thrust2force_B, thrust2torque_B)
[y, resnorm, ~, exitflag, output] = lsqnonneg(double([thrust2force_B; thrust2torque_B]), double([force_cmd;torque_cmd]));

iterations = output.iterations;


% sum1 = sum(y(1:6));
% sum2 = sum(y(7:12));
% sat_limit = .3;
% if any([sum1, sum2] > sat_limit)
%     sf = max([sum1, sum2])/sat_limit;
%     y = y./sf;
% end
%

== matlab function fam_force_allocation_module_lib/fam_force_allocation_module/calc_nozzle_thrust/latch_nozzle_thrust_matricies/MATLAB Function ==
  data: P_CG_B_B input size=[1 3]; force2thrust_B output; torque2thrust_B output; P_nozzle_B_B input; nozzle_orientations input; thrust2force_B output; thrust2torque_B output; forcetorque2thrust_B output
function [force2thrust_B, torque2thrust_B, thrust2force_B, thrust2torque_B, forcetorque2thrust_B] = calc_thrust_matricies(P_CG_B_B, P_nozzle_B_B, nozzle_orientations)
%#codegen

%NOTE: if number of nozzles change, must change this hard coded '12' below
nozzle_moment_arm       = P_nozzle_B_B - repmat(P_CG_B_B,12,1);                 %[m] Distance from nozzles to CG

thrust2torque_B         = -cross(nozzle_moment_arm, nozzle_orientations,2)';   %[-] Converts a nozzle thrust into resulting body torques
torque2thrust_B         = pinv(thrust2torque_B);                               %[-] Converts body torques into nozzle thrust
thrust2force_B          = -nozzle_orientations';                               %[-] Converts a nozzle thrust into resulting body forces
force2thrust_B          = pinv(thrust2force_B);                                %[-] Converts body forces into nozzle thrust

forcetorque2thrust_B = pinv([thrust2force_B;thrust2torque_B]);

end
